simulink library "Steer_DragLink"  (R2022a)
settings: Solver=VariableStepAuto  StartTime=0.0  StopTime=10.0  RelTol=1e-3
undefined symbols (not defined in the file): VDatabase, Visual
libraries: Steer_DragLink_Cross_Actuator x1, Steer_DragLink_Cross_WheelDriven x1, Vehicle_Inputs x1
Description:
  | Component of Simscape Vehicle Templates Library
  | 
  | Copyright 2018-2024 The MathWorks, Inc.
settings Model: Creator=smiller  LastModifiedBy=smiller
settings SolverCC: AlgebraicLoopSolver=TrustRegion
settings DataIOCC: ReturnWorkspaceOutputs=off
settings DebuggingCC: UnconnectedInputMsg=warning  UnconnectedOutputMsg=warning  UnconnectedLineMsg=warning  ArithmeticOperatorsInVariantConditions=warning
settings SFSimCC: CustomCodeUndefinedFunction=UseInterfaceOnly
settings RTWCC: DLArmComputeVersion=19.05

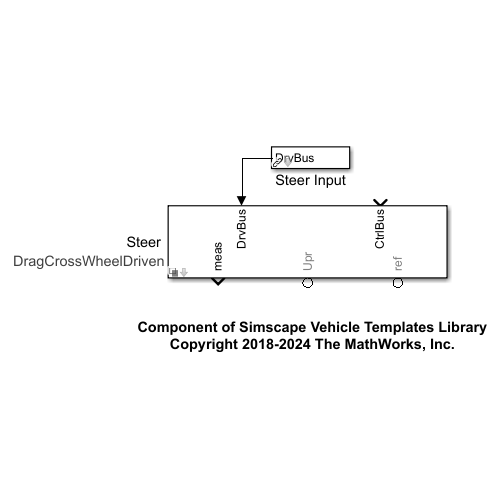
[thumbnail: Simulink's stored preview of the top-level diagram]
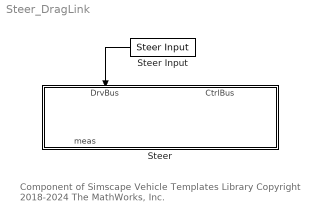
== system Steer_DragLink ==
  note: Component of Simscape Vehicle Templates Library
      | Copyright 2018-2024 The MathWorks, Inc.
  Steer : Subsystem  Variant=on  VariantControlMode=label  VariantControl=Steer  LabelModeActiveChoice=DragCrossWheelDriven  mask(Steering Systems, Drag Link){Steer=VDatabase.Steer.CrossWDriven_SUV_Landy_f, VariantLabel=VDatabase.Steer.CrossWDriven_SUV_Landy_f.class.Value}
      mask prompts: Steer "Steer Parameters"; VariantLabel "Variant Label"
      mask help: Steering system with drag link connection to suspension. Variant label selects active variant.
      mask init:
      | curblk = gcb;
      | 
      | % Set variant for this block 
      | set_param(curblk,'LabelModeActiveChoice',VariantLabel);
      settings: AttributesFormatString=%<ActiveVariant>
      mask Display: disp(' ');
  Steer Input : Vehicle_Inputs/DrvBus/Steer Input  popup_steer_input=Sequence
  wires:
  Steer Input/1 -> Steer/1(DrvBus)

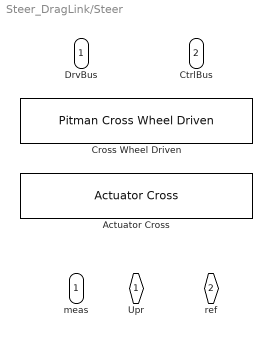
== system Steer_DragLink/Steer ==
  DrvBus : Inport
  CtrlBus : Inport  Port=2
  Actuator Cross : Steer_DragLink_Cross_Actuator/Actuator Cross  Tag=PublishSubsystem  VariantControl=DragCrossActuator  hp_actuator_mt=Steer.Actuator.sMount.Value  hp_drag_upr=Steer.DragLink.sUpright.Value  actuator_mass=Steer.Actuator.m.Value  drag_mass=Steer.DragLink.m.Value  actuator_filter=1/Steer.Actuator.fActuatorCutoff.Value  actuator_stroke=Steer.Actuator.xStroke.Value  clr_drag=Visual.Pushrod.clr  opc_drag=Visual.part.opc  radius_drag=Visual.Pushrod.rad  clr_actuator=Visual.Actuator.clr  opc_actuator=Visual.part.opc*0.7  rad_actuator=Visual.Pushrod.rad*2  clr_connhp=Visual.hp.clr  opc_connhp=Visual.hp.opc  size_connhp=Visual.hp.rad
  Cross Wheel Driven : Steer_DragLink_Cross_WheelDriven/Pitman Cross Wheel Driven  Tag=PublishSubsystem  VariantControl=DragCrossWheelDriven  hp_wheel=Steer.Wheel.sMount.Value  wheel_axis_incl=Steer.Wheel.aAxis.Value  hp_pitman_mt=Steer.PitmanArm.sMount.Value  hp_pitman_drag=Steer.DragLink.sPitmanArm.Value  hp_drag_upr=Steer.DragLink.sUpright.Value  Wheel=Steer.Wheel  len_sha_u=Steer.Shaft_Upper.xLength.Value  sha_u_mass=Steer.Shaft_Upper.m.Value  sha_i_mass=Steer.Shaft_Intermediate.m.Value  len_sha_l=Steer.Shaft_Lower.xLength.Value  sha_l_mass=Steer.Shaft_Lower.m.Value  pitman_mass=Steer.PitmanArm.m.Value  drag_mass=Steer.DragLink.m.Value  whl2steer_filter=1/Steer.Wheel.fActuatorCutoff.Value  nGear=Steer.Gear.nRatio.Value  clr_shaft=Visual.SteeringShafts.clr  opc_shaft=Visual.part.opc  size_shaft=Visual.SteeringShafts.rad  clr_rod=Visual.SteeringPinion.clr  opc_rod=Visual.part.opc  radius_rod=Visual.SteeringShafts.rad  clr_drag=Visual.TrackRod.clr  opc_drag=Visual.part.opc  radius_drag=Visual.TrackRod.rad  clr_connhp=Visual.hp.clr  opc_connhp=Visual.hp.opc  size_connhp=Visual.hp.rad  clr_wheel=Visual.SteeringWheel.clr  opc_wheel=Visual.part.opc  DriverHuman=VDatabase.DriverHuman.SUV_Landy
  " Upr" : PMIOPort  Side=Right
  " ref" : PMIOPort  Port=2  Side=Right
  " meas" : Outport  VectorParamsAs1DForOutWhenUnconnected=off
